simulink model "Regressor"  (R2020a)
settings: Solver=FixedStepAuto  StartTime=0.0  StopTime=10.0  FixedStep=DT  RelTol=1e-3
values from neighbouring files (symbols this model uses):
  T_s = 0.1    [run_Top_Model.m]
undefined symbols (not defined in the file or in its folder): DiscIntNeverNeededParam, forTime, magnitude, T_f, T_mean
libraries: dspmtrx3 x1, ctrlSharedLib x1
settings Model: Creator=lpwoolcock  LastModifiedBy=arthu

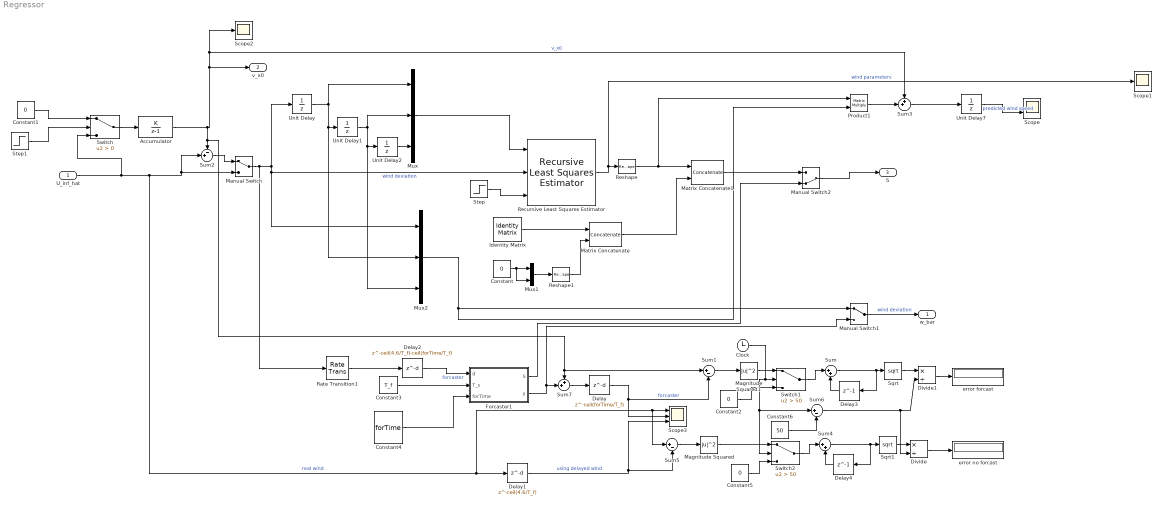
== system Regressor ==
  U_inf_hat : Inport  SampleTime=T_s
  Accumulator : DiscreteIntegrator  IntegratorMethod=Accumulation: Forward Euler  gainval=T_s/T_mean  SampleTime=T_s  ICPrevOutput=DiscIntNeverNeededParam  ICPrevScaledInput=DiscIntNeverNeededParam
  Clock : Clock
  Constant{,1..2,5} (4 alike) : Constant  Value=0
  Constant3 : Constant  Value=T_f
  Constant4 : Constant  Value=forTime
  Constant6 : Constant  Value=50
  Delay : Delay  DelayLength=ceil(forTime/T_f)  InitialCondition=0  SampleTime=T_f
  Delay1 : Delay  DelayLength=ceil(4.6/T_f)  InitialCondition=0  SampleTime=T_f
  Delay2 : Delay  DelayLength=ceil(4.6/T_f)-ceil(forTime/T_f)  InitialCondition=0  SampleTime=T_f
  Delay3 : Delay  DelayLength=1  InitialCondition=0
  Delay4 : Delay  DelayLength=1  InitialCondition=0
  Divide : Product  Inputs=*/
  Divide1 : Product  Inputs=*/
  Forcaster1 : MATLAB Function  TreatAsAtomicUnit=on
  Identity Matrix : dspmtrx3/Identity Matrix  Inherit=off  N=2  Ts=T_s  dataType=double  isSigned=on  wordLen=16  udDataType=sfix(16)  fracBitsMode=Best precision  numFracBits=15  OutDataTypeStr=double  LastOutDataTypeStr=double
  Magnitude Squared : Math  Operator=magnitude^2  SaturateOnIntegerOverflow=on
  Magnitude Squared1 : Math  Operator=magnitude^2  SaturateOnIntegerOverflow=on
  Manual Switch : ManualSwitch
  Manual Switch1 : ManualSwitch
  Manual Switch2 : ManualSwitch  CurrentSetting=0
  Matrix Concatenate : Concatenate  Mode=Multidimensional array  ConcatenateDimension=2
  Matrix Concatenate1 : Concatenate  Mode=Multidimensional array
  Mux : Mux  Inputs=3
  Mux1 : Mux  Inputs=2
  Mux2 : Mux  Inputs=3
  Product1 : Product  Multiplication=Matrix(*)
  Rate Transition1 : RateTransition  Deterministic=off  OutPortSampleTime=T_f
  Recursive Least Squares Estimator : ctrlSharedLib/Recursive Least Squares Estimator  InitialEstimateSource=None  InitialParameterData=3  P0=1e4  InitialRegressors=0  InitialOutputs=0  History=Infinite  WindowLength=200  EstimationMethod=Forgetting Factor  AdaptationParameter=0.9  HasTimeVaryingAdaptationParameter=off  NormalizationBias=eps  OutputError=off  OutputP=off  AddEnablePort=off  ExternalReset=Rising  InputProcessing=Sample-based  Ts=-1
      settings: SourceProductBaseCode=CT,ID
  Reshape : Reshape  OutputDimensionality=Row vector (2-D)
  Reshape1 : Reshape  OutputDimensionality=Column vector (2-D)
  Scope : Scope  NumInputPorts=2
  Scope1 : Scope
  Scope2 : Scope
  Scope3 : Scope  NumInputPorts=3
  Sqrt : Sqrt  SaturateOnIntegerOverflow=on
  Sqrt1 : Sqrt  SaturateOnIntegerOverflow=on
  Step : Step  Time=T_mean  SampleTime=T_s
  Step1 : Step  Time=T_mean  SampleTime=T_s
  Sum : Sum  Inputs=|++
  Sum1 : Sum  Inputs=|+-
  Sum2 : Sum  Inputs=-+|
  Sum3 : Sum  Inputs=++|
  Sum4 : Sum  Inputs=|++
  Sum5 : Sum  Inputs=|+-
  Sum6 : Sum  Inputs=|+-
  Sum7 : Sum  Inputs=++|
  Switch : Switch  Criteria=u2 > Threshold
  Switch1 : Switch  Criteria=u2 > Threshold  Threshold=50
  Switch2 : Switch  Criteria=u2 > Threshold  Threshold=50
  Unit Delay{,1..2,7} (4 alike) : UnitDelay  SampleTime=-1  HasFrameUpgradeWarning=on
  error forcast : Display
  error no forcast : Display
  w_bar : Outport  SampleTime=T_s
  v_x0 : Outport  Port=2  SampleTime=T_s
  S : Outport  Port=3  SampleTime=T_s
  wires:
  Matrix Concatenate/1 -> Matrix Concatenate1/2
  Mux/1 -> Recursive Least Squares Estimator/1
  Unit Delay2/1 -> Mux/3
  Matrix Concatenate1/1 -> Manual Switch2/1
  Reshape/1 -> Product1/1, Matrix Concatenate1/1
  Constant/1 -> Mux1/2, Mux1/1
  Reshape1/1 -> Matrix Concatenate/2
  Mux1/1 -> Reshape1/1
  Unit Delay1/1 -> Mux/2, Mux2/3, Unit Delay2/1
  Recursive Least Squares Estimator/1 -> Scope1/1, Reshape/1  "wind parameters"
  Identity Matrix/1 -> Matrix Concatenate/1
  Unit Delay/1 -> Mux/1, Mux2/2, Unit Delay1/1
  Mux2/1 -> Manual Switch1/1, Product1/2
  Unit Delay7/1 -> Scope/2  "predicted wind speed"
  Manual Switch/1 -> Rate Transition1/1, Mux2/1, Recursive Least Squares Estimator/2, Unit Delay/1  "wind deviation"
  Sum3/1 -> Unit Delay7/1
  Step/1 -> Recursive Least Squares Estimator/3
  Step1/1 -> Switch/2
  Constant1/1 -> Switch/1
  Switch/1 -> Accumulator/1
  Accumulator/1 -> Sum1/1, Sum7/1, Sum2/1, v_x0/1, Sum3/1, Scope2/1  "v_x0"
  Product1/1 -> Sum3/2
  Sum2/1 -> Manual Switch/1
  Constant3/1 -> Forcaster1/2(T_s)
  Forcaster1/2(y) -> Sum7/2, Manual Switch1/2
  Delay/1 -> Sum1/2, Scope3/2  "forcaster"
  Constant4/1 -> Forcaster1/3(forTime)
  U_inf_hat/1 -> Sum5/1, Scope3/1, Delay1/1, Manual Switch/2, Sum2/2, Switch/3  "real wind"
  Delay1/1 -> Scope3/3, Sum5/2  "using delayed wind"
  Delay2/1 -> Forcaster1/1(d)  "forcaster"
  Sum1/1 -> Magnitude Squared1/1
  Delay3/1 -> Sum/2
  Sum/1 -> Sqrt/1, Delay3/1
  Magnitude Squared1/1 -> Switch1/1
  Switch1/1 -> Sum/1
  Constant2/1 -> Switch1/3
  Switch2/1 -> Sum4/1
  Clock/1 -> Sum6/1, Switch2/2, Switch1/2
  Magnitude Squared/1 -> Switch2/1
  Sum5/1 -> Magnitude Squared/1
  Delay4/1 -> Sum4/2
  Constant5/1 -> Switch2/3
  Sum4/1 -> Sqrt1/1, Delay4/1
  Sqrt1/1 -> Divide/1
  Divide/1 -> error no forcast/1
  Sqrt/1 -> Divide1/1
  Divide1/1 -> error forcast/1
  Constant6/1 -> Sum6/2
  Sum6/1 -> Divide/2, Divide1/2
  Manual Switch1/1 -> w_bar/1  "wind deviation"
  Rate Transition1/1 -> Delay2/1
  Sum7/1 -> Delay/1
  Manual Switch2/1 -> S/1
  Forcaster1/1(S) -> Manual Switch2/2

== matlab function Regressor/Forcaster1 ==
  data: S output; d input; y output; T_s input; forTime input
%This function uses recursive least squares and numerical integration 
%to forcast the wind  signal.
%USAGE: d last known windspeed
%T_s the sample rate
%forTime how far in the future the output is
%returns y estimate of the windspeed at t+forTime
function [S,y]= forcaster_2(d,T_s,forTime)


%Set Forcast time in init callback

num_for = ceil(forTime/T_s);    %number of samples forcast
order = 3;                      %order of regression
delta = 1;                      %P initialisation param
lambda = 0.99;                  %forgetting factor
sat_limit = 28;                 %saturation limit of output.(poor choice of delta/poor paraeter choice can cause big spikes)

%set up registers
persistent U;
if(isempty(U))
   U = zeros(order,1);
end

persistent Z;
if(isempty(Z))
   Z = zeros(order,1);
end

persistent P;
if(isempty(P)) 
    P = eye(size(U,1))*delta;
end


%recursive least squares
K = P*U/(lambda+U'*P*U);
zeta = d-Z'*U;
Z = Z+K*zeta;
P = P/lambda-K*U'*P/lambda;

%update register
U(2:end,1) = U(1:end-1,1);
U(1,1) = d; 

S = [Z';eye(order-1) zeros(order-1,1)];
Y = (S^num_for)*U;
y = Y(1,1);
if(y>sat_limit) %saturation
    y(1,1) = sat_limit;
end
if(y(1,1)<0)
   y(1,1)=0; 
end
end
